simulink model "TASK1_walking_sideways"  (R2022b)
settings: Solver=VariableStepAuto  StartTime=0.0  StopTime=8  RelTol=1e-3
values from neighbouring files (symbols this model uses):
  m = 12    [MPC_Controller.m]    (also in QP_Controller.m; TASK1_rotating_mpc.m; TASK1_walking_backward_mpc.m; TASK1_walking_forward_mpc.m)
  N = 10    [MPC_Controller.m]
undefined symbols (not defined in the file or in its folder): TASK1_walking_sideways_mpc, X, Y, Z
libraries: sm_lib x188, nesl_utility x122, simulink x1
(part 6 of 6)

== matlab function TASK1_walking_sideways/Walk Controller/Swing Controller1/Calculate Swing Leg Velocity ==
  data: FL_vx output; FL_vy output; v_com_vec input; FL_vz output; T_stance input; v_desired input; hip_data input; FR_foot_pos input; FL_foot_pos input; RL_foot_pos input; FR_vx output; FR_vy output; FR_vz output; RL_vx output; RL_vy output; RL_vz output; RR_vx output; RR_vy output; RR_vz output; FR_foot_init output; RR_foot_pos input; FL_foot_init output; RL_foot_init output; RR_foot_init output; t input
function [FL_vx,FL_vy,FL_vz,FR_vx,FR_vy,FR_vz,RL_vx,RL_vy,RL_vz,RR_vx,RR_vy,RR_vz,FR_foot_init,FL_foot_init,RL_foot_init,RR_foot_init] = fcn(v_com_vec,T_stance,v_desired,hip_data,FR_foot_pos,FL_foot_pos,RL_foot_pos,RR_foot_pos,t)

z_height = 0.1; 

FL_hip_pos = hip_data(1:3);
FR_hip_pos = hip_data(4:6);
RL_hip_pos = hip_data(7:9);
RR_hip_pos = hip_data(10:12);
FR_foot_init = FR_foot_pos;
FL_foot_init = FL_foot_pos;
RL_foot_init = RL_foot_pos;
RR_foot_init = RR_foot_pos;


steps = 0:T_stance:10; 
index = discretize(t,steps); 

% Find K_step - this value can be tuned with z_com_desired
z_com_desired = 0.3;
g = 9.81;
K_step = sqrt(z_com_desired/g);

%% FL
% Find P_foot_desired - FL
FL_hip_pos(3) = 0;
FL_p_foot_desired_end = FL_hip_pos+(T_stance/2)*v_desired+K_step*(v_com_vec-v_desired);
FL_p_foot_desired_end(3) = 0;

% Create Trajectory 
half_step = (FL_p_foot_desired_end - FL_foot_pos)/2+[0;0;z_height];
half_step_time = T_stance/2;
v = half_step/half_step_time;

FL_vx = v(1);
FL_vy = v(2);
FL_vz = v(3);

%% FR
% Find P_foot_desired - FR
FR_hip_pos(3) = 0;
FR_p_foot_desired_end = FR_hip_pos+(T_stance/2)*v_desired+K_step*(v_com_vec-v_desired);
FR_p_foot_desired_end(3) = 0;

% Create Trajectory 
half_step = (FR_p_foot_desired_end - FR_foot_pos)/2+[0;0;z_height];
half_step_time = T_stance/2;
v = half_step/half_step_time;

FR_vx = v(1);
FR_vy = v(2);
FR_vz = v(3);

%% RL
% Find P_foot_desired - RL
RL_hip_pos(3) = 0;
RL_p_foot_desired_end = RL_hip_pos+(T_stance/2)*v_desired+K_step*(v_com_vec-v_desired);
RL_p_foot_desired_end(3) = 0;

% Create Trajectory 
half_step = (RL_p_foot_desired_end - RL_foot_pos)/2+[0;0;z_height];
half_step_time = T_stance/2;
v = half_step/half_step_time;

RL_vx = v(1);
RL_vy = v(2);
RL_vz = v(3);


%% RR
% Find P_foot_desired - RR
RR_hip_pos(3) = 0;
RR_p_foot_desired_end = RR_hip_pos+(T_stance/2)*v_desired+K_step*(v_com_vec-v_desired);
RR_p_foot_desired_end(3) = 0;

% Create Trajectory 
half_step = (RR_p_foot_desired_end - RR_foot_pos)/2+[0;0;z_height];
half_step_time = T_stance/2;
v = half_step/half_step_time;

RR_vx = v(1);
RR_vy = v(2);
RR_vz = v(3);

== matlab function TASK1_walking_sideways/Walk Controller/Swing Controller1/Create Forces for Swing Leg ==
  data: FL_vx input; F_swing output; FL_vy input; FL_vz input; FR_vx input; FR_vy input; FR_vz input; RL_vx input; RL_vy input; RL_vz input; RR_vx input; RR_vy input; RR_vz input; T_stance input; FL_foot_pos input; FR_foot_pos input; RL_foot_pos input; RR_foot_pos input; FL_foot_vel input; FR_foot_vel input; RL_foot_vel input; RR_foot_vel input; init_FR_pos input; init_FL_pos input; init_RL_pos input; init_RR_pos input; t input; FR_p_desired output; FR_p_foot output
function [F_swing,FR_p_desired,FR_p_foot]  = fcn(FL_vx,FL_vy,FL_vz,FR_vx,FR_vy,FR_vz,RL_vx,RL_vy,RL_vz,RR_vx,RR_vy,RR_vz,T_stance,FL_foot_pos,FR_foot_pos,RL_foot_pos,RR_foot_pos,FL_foot_vel,FR_foot_vel,RL_foot_vel,RR_foot_vel,init_FR_pos,init_FL_pos,init_RL_pos,init_RR_pos,t)

% These are the desired velocity values calculated from the previous block
% These are the desired velocity for each foot position through the swing
FL_v_desired = [FL_vx;FL_vy;FL_vz];
FR_v_desired = [FR_vx;FR_vy;FR_vz];
RL_v_desired = [RL_vx;RL_vy;RL_vz];
RR_v_desired = [RR_vx;RR_vy;RR_vz];

z_height = 0.1; 
% These are the actual current foot position and velocity - these update
% continously
FL_p_foot = FL_foot_pos(1:3);
FL_v_foot = FL_foot_vel(1:3);
FR_p_foot = FR_foot_pos(1:3);
FR_v_foot = FR_foot_vel(1:3);
RL_p_foot = RL_foot_pos(1:3);
RL_v_foot = RL_foot_vel(1:3);
RR_p_foot = RR_foot_pos(1:3);
RR_v_foot = RR_foot_vel(1:3);

steps = 0:T_stance:10; 

if t <= 0.2 
    FL_px = 0;
    FL_py = 0; 
    FL_pz = 0;
    FR_px = 0;
    FR_py = 0; 
    FR_pz = 0; 
    RL_px = 0;
    RL_py = 0; 
    RL_pz = 0; 
    RR_px = 0;
    RR_py = 0; 
    RR_pz = 0; 
    
else
    step_index = discretize(t,steps);
    delta_t = t-steps(step_index);
   
    % Find the DELTA desired position of the foot using the time
    % This wil be added to the intitial foot position
    FL_px = FL_vx*delta_t; 
    FL_py = FL_vy*delta_t; 
    FL_pz = FL_vz*delta_t;
    FR_px = FR_vx*delta_t; 
    FR_py = FR_vy*delta_t; 
    FR_pz = FR_vz*delta_t; 
    RL_px = RL_vx*delta_t; 
    RL_py = RL_vy*delta_t; 
    RL_pz = RL_vz*delta_t; 
    RR_px = RR_vx*delta_t; 
    RR_py = RR_vy*delta_t; 
    RR_pz = RR_vz*delta_t; 
    if FL_pz > z_height
        FL_pz = z_height-FL_vz*(delta_t-T_stance/2);
        FL_v_desired(3) = -FL_v_desired(3);
    end
    if FR_pz > z_height
        FR_pz = z_height-FR_vz*(delta_t-T_stance/2);
        FR_v_desired(3) = -FR_v_desired(3);
    end
    if RL_pz > z_height
        RL_pz = z_height-RL_vz*(delta_t-T_stance/2);
        RL_v_desired(3) = -RL_v_desired(3);
    end
    if RR_pz > z_height
        RR_pz = z_height-RR_vz*(delta_t-T_stance/2);
        RR_v_desired(3) = -RR_v_desired(3);
    end

end

z_offset = 0.01;
% Foot pos desired at time t 
FL_p_desired = [init_FL_pos(1); init_FL_pos(2)+0.08; 0] + [FL_px;FL_py;FL_pz];
FR_p_desired = [init_FR_pos(1); init_FR_pos(2)-0.08; 0] + [FR_px;FR_py;FR_pz];
RL_p_desired = [init_RL_pos(1); init_RL_pos(2)+0.08; 0] + [RL_px;RL_py;RL_pz];
RR_p_desired = [init_RR_pos(1); init_RR_pos(2)-0.08; 0] + [RR_px;RR_py;RR_pz];

FL_p_foot = FL_p_foot - [0;0;z_offset];
FR_p_foot = FR_p_foot - [0;0;z_offset];
RL_p_foot = RL_p_foot - [0;0;z_offset];
RR_p_foot = RR_p_foot - [0;0;z_offset];

% Find the force using a PD controller - FL
KP = [400;400;400]; 
KD = [10;10;10]; 
F_swing_FL = KP.*(FL_p_desired-FL_p_foot)+KD.*(FL_v_desired-FL_v_foot);
F_swing_FR = KP.*(FR_p_desired-FR_p_foot)+KD.*(FR_v_desired-FR_v_foot);
F_swing_RL = KP.*(RL_p_desired-RL_p_foot)+KD.*(RL_v_desired-RL_v_foot);
F_swing_RR = KP.*(RR_p_desired-RR_p_foot)+KD.*(RR_v_desired-RR_v_foot);

F_swing = [F_swing_FL;F_swing_RL; F_swing_FR; F_swing_RR];

== matlab function TASK1_walking_sideways/Walk Controller/MATLAB Function ==
  data: P input; pos_d output; v_d input
function pos_d = fcn(P,v_d)
dt = 0.05;
pos_d = P(2)+ 10*dt*v_d(2);

== matlab function TASK1_walking_sideways/MATLAB Function ==
  data: t input; FL output; torques_stand input; torques_walk input; RL output; FR output; RR output
function [FL, RL, FR, RR] = fcn(t, torques_stand, torques_walk)
%#codegen
if t < 1
    FL = torques_stand(1:3);
    RL = torques_stand(4:6);
    FR = torques_stand(7:9);
    RR = torques_stand(10:12);
else
    FL = torques_walk(1:3);
    RL = torques_walk(4:6);
    FR = torques_walk(7:9);
    RR = torques_walk(10:12);
end

== matlab function TASK1_walking_sideways/Walk Controller/Convert Forces to Torque1/Force to Torque ==
  data: F input; Tau_RR output; RR_ang_vec input; RL_ang_vec input; FL_ang_vec input; FR_ang_vec input; Tau_FR output; Tau_FL output; Tau_RL output
function [Tau_RR,Tau_FR,Tau_FL,Tau_RL]= fcn(F,RR_ang_vec,RL_ang_vec,FL_ang_vec,FR_ang_vec)
    % TODO - Convert forces to torques using the inverse jacobian
    % Get forces from the force vector 
    % NOTE - VERIFY THAT THESE ARE THE CORRECT VECTORS (I am unsure)
    F_FL = F(1:3);
    F_RL = F(4:6);
    F_FR = F(7:9);
    F_RR = F(10:12);

    l1=0.045; % hip length
    l2=0.2; % thigh length
    l3=0.2; % calf length
    

    %% Calculate the force for the RR leg - NOTE: The right legs have the
    % same jacobians
    q = RR_ang_vec; %
    leg = 4;
  
    if leg==1 || leg==3 % left leg has sideSign 1
        sideSign=1;
    else
        sideSign=-1; % right leg has sideSign -1
    end
    s1=sin(q(1)); % for hip joint
    s2=sin(q(2)); % for thigh joint
    s3=sin(q(3)); % for calf joint

    c1=cos(q(1)); % for hip joint
    c2=cos(q(2)); % for thigh joint
    c3=cos(q(3)); % for calf joint
    
    c23=c2*c3-s2*s3;
    s23=s2*c3+c2*s3;
    J = eye(3);
    J(1,1)=0;
    J(2,1)=-sideSign*l1*s1+l2*c2*c1+l3*c23*c1;
    J(3,1)=sideSign*l1*c1+l2*c2*s1+l3*c23*s1;
    
    J(1,2)=-l3*c23-l2*c2;
    J(2,2)=-l2*s2*s1-l3*s23*s1;
    J(3,2)=l2*s2*c1+l3*s23*c1;

    J(1,3)=-l3*c23;
    J(2,3)=-l3*s23*s1;
    J(3,3)=l3*s23*c1;
    
    inJ_R_RR = transpose(J);
    Tau_RR = -inJ_R_RR*F_RR;

  
    %% Calculate the force for the FR leg - NOTE: The right legs have the
    % same jacobians
    q = FR_ang_vec; %
    leg = 2;
  
    if leg==1 || leg==3 % left leg has sideSign 1
        sideSign=1;
    else
        sideSign=-1; % right leg has sideSign -1
    end
    s1=sin(q(1)); % for hip joint
    s2=sin(q(2)); % for thigh joint
    s3=sin(q(3)); % for calf joint

    c1=cos(q(1)); % for hip joint
    c2=cos(q(2)); % for thigh joint
    c3=cos(q(3)); % for calf joint
    
    c23=c2*c3-s2*s3;
    s23=s2*c3+c2*s3;

    J(1,1)=0;
    J(2,1)=-sideSign*l1*s1+l2*c2*c1+l3*c23*c1;
    J(3,1)=sideSign*l1*c1+l2*c2*s1+l3*c23*s1;
    
    J(1,2)=-l3*c23-l2*c2;
    J(2,2)=-l2*s2*s1-l3*s23*s1;
    J(3,2)=l2*s2*c1+l3*s23*c1;

    J(1,3)=-l3*c23;
    J(2,3)=-l3*s23*s1;
    J(3,3)=l3*s23*c1;

    inJ_R_FR = transpose(J);
    Tau_FR = -inJ_R_FR*F_FR;

    %% Calculate the force for the FL leg - NOTE: The right legs have the
    % same jacobians
    q = FL_ang_vec; %
    leg = 1;
  
    if leg==1 || leg==3 % left leg has sideSign 1
        sideSign=1;
    else
        sideSign=-1; % right leg has sideSign -1
    end
    s1=sin(q(1)); % for hip joint
    s2=sin(q(2)); % for thigh joint
    s3=sin(q(3)); % for calf joint

    c1=cos(q(1)); % for hip joint
    c2=cos(q(2)); % for thigh joint
    c3=cos(q(3)); % for calf joint
    
    c23=c2*c3-s2*s3;
    s23=s2*c3+c2*s3;

    J(1,1)=0;
    J(2,1)=-sideSign*l1*s1+l2*c2*c1+l3*c23*c1;
    J(3,1)=sideSign*l1*c1+l2*c2*s1+l3*c23*s1;
    
    J(1,2)=-l3*c23-l2*c2;
    J(2,2)=-l2*s2*s1-l3*s23*s1;
    J(3,2)=l2*s2*c1+l3*s23*c1;

    J(1,3)=-l3*c23;
    J(2,3)=-l3*s23*s1;
    J(3,3)=l3*s23*c1;

    inJ_R_FL = transpose(J);
    Tau_FL = -inJ_R_FL*F_FL;


    %% Calculate the force for the RL leg - NOTE: The right legs have the
    % same jacobians
    q = RL_ang_vec; %
    leg = 3;
  
    if leg==1 || leg==3 % left leg has sideSign 1
        sideSign=1;
    else
        sideSign=-1; % right leg has sideSign -1
    end
    s1=sin(q(1)); % for hip joint
    s2=sin(q(2)); % for thigh joint
    s3=sin(q(3)); % for calf joint

    c1=cos(q(1)); % for hip joint
    c2=cos(q(2)); % for thigh joint
    c3=cos(q(3)); % for calf joint
    
    c23=c2*c3-s2*s3;
    s23=s2*c3+c2*s3;

    J(1,1)=0;
    J(2,1)=-sideSign*l1*s1+l2*c2*c1+l3*c23*c1;
    J(3,1)=sideSign*l1*c1+l2*c2*s1+l3*c23*s1;
    
    J(1,2)=-l3*c23-l2*c2;
    J(2,2)=-l2*s2*s1-l3*s23*s1;
    J(3,2)=l2*s2*c1+l3*s23*c1;

    J(1,3)=-l3*c23;
    J(2,3)=-l3*s23*s1;
    J(3,3)=l3*s23*c1;

    inJ_R_RL = transpose(J);
    Tau_RL = -inJ_R_RL*F_RL;

== matlab function TASK1_walking_sideways/Rear Left Leg/Separate Torques ==
  data: torque_vector input; hip_torque output; thigh_torque output; calf_torque output
function [hip_torque, thigh_torque, calf_torque] = fcn(torque_vector)

hip_torque = torque_vector(1);
thigh_torque = torque_vector(2);
calf_torque = torque_vector(3);

== matlab function TASK1_walking_sideways/Front Right Leg/Separate Torques ==
  data: torque_vector input; hip_torque output; thigh_torque output; calf_torque output
function [hip_torque, thigh_torque, calf_torque] = fcn(torque_vector)

hip_torque = torque_vector(1);
thigh_torque = torque_vector(2);
calf_torque = torque_vector(3);
